simulink model "radar_simulation"  (R2022a)
settings: Solver=VariableStepAuto  StartTime=0.0  StopTime=10  RelTol=1e-3
model workspace (MAT data in the model file):
  Antenna_Aperture = Simulink.Parameter
  Antenna_Aperture.Value = 2.025e-05
  Antenna_Aperture.DataType = 'auto'
  Antenna_Aperture.Min = 0
  Antenna_Aperture.DocUnits = 'm^2'
  Antenna_Aperture.Complexity = 'real'
  Antenna_Aperture.Dimensions = [1 1]
  Center_Frequency = Simulink.Parameter
  Center_Frequency.Value = 60000000000
  Center_Frequency.DataType = 'auto'
  Center_Frequency.Min = 60000000000
  Center_Frequency.Max = 64000000000
  Center_Frequency.DocUnits = 'Hz'
  Center_Frequency.Complexity = 'real'
  Center_Frequency.Dimensions = [1 1]
  Max_Range = Simulink.Parameter
  Max_Range.Value = 100
  Max_Range.DataType = 'auto'
  Max_Range.Min = 0
  Max_Range.DocUnits = 'm'
  Max_Range.Complexity = 'real'
  Max_Range.Dimensions = [1 1]
  Sample_Rate = Simulink.Parameter
  Sample_Rate.Value = 16000000
  Sample_Rate.DataType = 'auto'
  Sample_Rate.Min = 0
  Sample_Rate.DocUnits = 'Hz'
  Sample_Rate.Complexity = 'real'
  Sample_Rate.Dimensions = [1 1]
  Samples_Per_CPI = Simulink.Parameter
  Samples_Per_CPI.Value = Simulink.data.Expression
  Samples_Per_CPI.Value.ExpressionString = "Samples_Per_Sweep * Sweeps_Per_CPI"
  Samples_Per_CPI.DataType = 'auto'
  Samples_Per_CPI.Complexity = 'real'
  Samples_Per_CPI.Dimensions = -1
  Samples_Per_Sweep = Simulink.Parameter
  Samples_Per_Sweep.Value = Simulink.data.Expression
  Samples_Per_Sweep.Value.ExpressionString = "Sample_Rate * Sweep_Interval"
  Samples_Per_Sweep.DataType = 'auto'
  Samples_Per_Sweep.Complexity = 'real'
  Samples_Per_Sweep.Dimensions = -1
  Sweep_Bandwidth = Simulink.Parameter
  Sweep_Bandwidth.Value = 135000000
  Sweep_Bandwidth.DataType = 'auto'
  Sweep_Bandwidth.Min = 0
  Sweep_Bandwidth.DocUnits = 'Hz'
  Sweep_Bandwidth.Complexity = 'real'
  Sweep_Bandwidth.Dimensions = [1 1]
  Sweep_Interval = Simulink.Parameter
  Sweep_Interval.Value = 4.5e-05
  Sweep_Interval.DataType = 'auto'
  Sweep_Interval.DocUnits = 's'
  Sweep_Interval.Complexity = 'real'
  Sweep_Interval.Dimensions = [1 1]
  Sweeps_Per_CPI = Simulink.Parameter
  Sweeps_Per_CPI.Value = 128
  Sweeps_Per_CPI.DataType = 'auto'
  Sweeps_Per_CPI.Complexity = 'real'
  Sweeps_Per_CPI.Dimensions = [1 1]
undefined symbols (not defined in the file or in its folder): aperture2gain, freq2wavelen, physconst
libraries: phasedenvlib x4, phaseddetectlib x2, phasedtxrxlib x2, phasedwavlib x1
settings Model: SimulationMode=accelerator  Creator=mhatch  LastModifiedBy=mhatch
settings SolverCC: DecoupledContinuousIntegration=on  MinimalZcImpactIntegration=on
settings DebuggingCC: ReadBeforeWriteMsg=DisableAll  WriteAfterWriteMsg=DisableAll  WriteAfterReadMsg=DisableAll  MultiTaskDSMMsg=none  AllowSymbolicDim=off
settings ModelReferenceCC: UpdateModelReferenceTargets=IfOutOfDate
settings SFSimCC: SFSimEcho=off

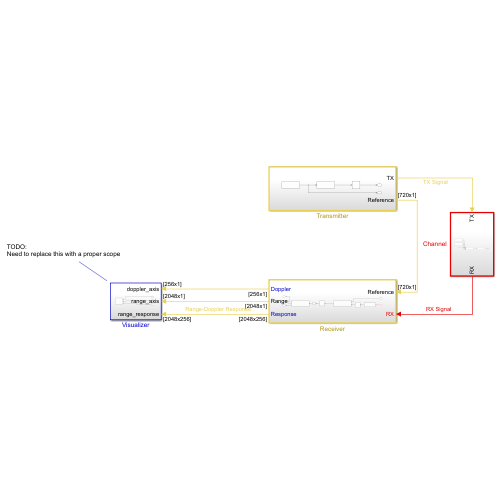
[thumbnail: Simulink's stored preview of the top-level diagram]
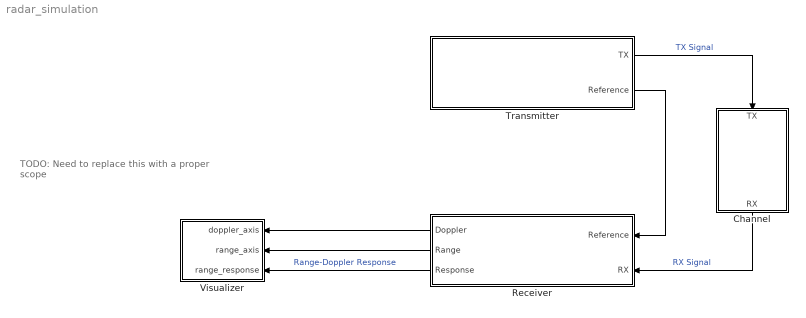
== system radar_simulation ==
  note: TODO:
      | Need to replace this with a proper scope
  Channel : Subsystem  TreatAsAtomicUnit=on
  Receiver : Subsystem  TreatAsAtomicUnit=on
  Transmitter : Subsystem  TreatAsAtomicUnit=on
  Visualizer : Subsystem
  wires:
  Transmitter/1(TX) -> Channel/1(TX)  "TX Signal"
  Channel/1(RX) -> Receiver/2(RX)  "RX Signal"
  Receiver/1(Doppler) -> Visualizer/1(doppler_axis)
  Receiver/2(Range) -> Visualizer/2(range_axis)
  Receiver/3(Response) -> Visualizer/3(range_response)  "Range-Doppler Response"
  Transmitter/2(Reference) -> Receiver/1(Reference)

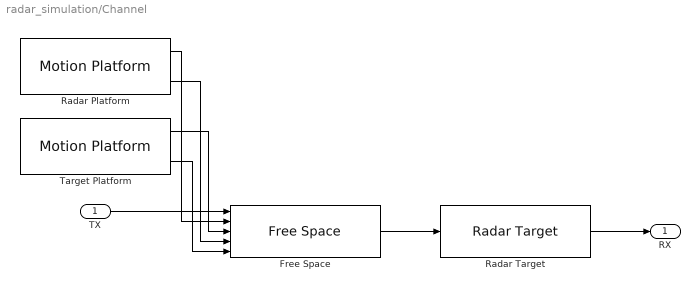
== system radar_simulation/Channel ==
  TX : Inport
  Free Space : phasedenvlib/Free Space  PropagationSpeed=physconst( 'LightSpeed' )  OperatingFrequency=Center_Frequency  TwoWayPropagation=on  SampleRateFromInputCheckbox=on  SampleRate=Sample_Rate  MaximumDistanceSource=Property  MaximumDistance=100  MaximumNumInputSamplesSource=Auto  MaximumNumInputSamples=1000  SimulateUsing=Code generation
      settings: SourceProductBaseCode=AR
  Radar Platform : phasedenvlib/Motion Platform  MotionModel=Velocity  InitialPosition=[ 0; 0; 0.5 ]  InitialVelocity=[ 0; 0; 0 ]  VelocitySource=Property  Velocity=[0; 0; 0]  AccelerationSource=Property  Acceleration=[0;0;0]  CustomTrajectory=[ 0, 0, 0, 0, 0, 0, 0; 1, 0, 0, 0, 0, 0, 0 ]  ScanMode=None  InitialScanAngle=0  AzimuthSpan=[ -60, 60 ]  AzimuthScanRate=10  InitialOrientationAxes=eye( 3 )  OrientationAxesOutputPort=off  ElapsedTimeSource=Auto  SampleRateFromInputCheckbox=on  SampleRate=1e6  SimulateUsing=Code generation
      settings: SourceProductBaseCode=AR
  Radar Target : phasedenvlib/Radar Target  EnablePolarization=off  Mode=Monostatic  MeanRCSSource=Property  ScatteringMatrixSource=Property  MeanRCS=min(pow2db(20), 0.1)  ScatteringMatrix=eye( 2 )  Model=Nonfluctuating  PropagationSpeed=physconst( 'LightSpeed' )  OperatingFrequency=Center_Frequency  SeedSource=Auto  Seed=0  SimulateUsing=Code generation
      settings: SourceProductBaseCode=AR
  Target Platform : phasedenvlib/Motion Platform  MotionModel=Velocity  InitialPosition=[ 20; 0; 0.5 ]  InitialVelocity=[ 0; 0; 0 ]  VelocitySource=Property  Velocity=[5; 0; 0]  AccelerationSource=Property  Acceleration=[0;0;0]  CustomTrajectory=[ 0, 0, 0, 0, 0, 0, 0; 1, 0, 0, 0, 0, 0, 0 ]  ScanMode=None  InitialScanAngle=0  AzimuthSpan=[ -60, 60 ]  AzimuthScanRate=10  InitialOrientationAxes=eye( 3 )  OrientationAxesOutputPort=off  ElapsedTimeSource=Auto  SampleRateFromInputCheckbox=on  SampleRate=1e6  SimulateUsing=Code generation
      settings: SourceProductBaseCode=AR
  RX : Outport
  wires:
  Radar Platform/1 -> Free Space/2
  Radar Platform/2 -> Free Space/4
  Target Platform/2 -> Free Space/5
  Target Platform/1 -> Free Space/3
  TX/1 -> Free Space/1
  Free Space/1 -> Radar Target/1
  Radar Target/1 -> RX/1

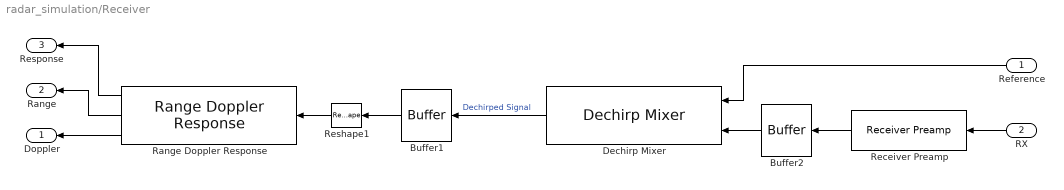
== system radar_simulation/Receiver ==
  Reference : Inport
  RX : Inport  Port=2
  Buffer1 : Buffer  N=Samples_Per_CPI  OutputFrames=off
  Buffer2 : Buffer  N=Samples_Per_Sweep  OutputFrames=off
  Dechirp Mixer : phaseddetectlib/Dechirp Mixer
      settings: SourceProductBaseCode=AR
  Range Doppler Response : phaseddetectlib/Range Doppler Response  RangeMethod=FFT  PropagationSpeed=physconst( 'lightspeed' )  SampleRateFromInputCheckbox=off  SampleRate=Sample_Rate  SweepSlope=Sweep_Bandwidth / Sweep_Interval  DechirpInput=off  RangeFFTLengthSource=Property  RangeFFTLength=2048  RangeWindow=None  RangeSidelobeAttenuation=30  CustomRangeWindow=@hamming  ReferenceRangeCentered=on  ReferenceRange=0  MaximumNumInputSamplesSource=Auto  MaximumNumInputSamples=100  PRFSource=Auto  PRF=10e3  DopplerFFTLengthSource=Property  DopplerFFTLength=256  DopplerWindow=None  DopplerSidelobeAttenuation=30  CustomDopplerWindow=@hamming  DopplerOutput=Speed  OperatingFrequency=Center_Frequency  SimulateUsing=Code generation
      settings: SourceProductBaseCode=AR
  Receiver Preamp : phasedtxrxlib/Receiver Preamp  Gain=15 + aperture2gain(Antenna_Aperture, freq2wavelen(Center_Frequency, physconst( 'LightSpeed')))  LossFactor=0  NoiseMethod=Noise temperature  NoiseFigure=4.5  ReferenceTemperature=290  SampleRateFromInputCheckbox=on  SampleRate=1e6  NoisePower=0  EnableInputPort=off  PhaseNoiseInputPort=off  SeedSource=Auto  Seed=0  SimulateUsing=Code generation
      settings: SourceProductBaseCode=AR
  Reshape1 : Reshape  OutputDimensionality=Customize  OutputDimensions=[Samples_Per_Sweep Sweeps_Per_CPI]
  Doppler : Outport
  Range : Outport  Port=2
  Response : Outport  Port=3
  wires:
  Buffer1/1 -> Reshape1/1
  Reference/1 -> Dechirp Mixer/1
  RX/1 -> Receiver Preamp/1
  Reshape1/1 -> Range Doppler Response/1
  Dechirp Mixer/1 -> Buffer1/1  "Dechirped Signal"
  Buffer2/1 -> Dechirp Mixer/2
  Receiver Preamp/1 -> Buffer2/1
  Range Doppler Response/3 -> Doppler/1
  Range Doppler Response/1 -> Response/1
  Range Doppler Response/2 -> Range/1

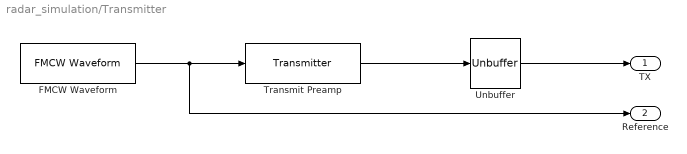
== system radar_simulation/Transmitter ==
  FMCW Waveform : phasedwavlib/FMCW Waveform  SampleRate=Sample_Rate  SweepTime=Sweep_Interval  SweepBandwidth=Sweep_Bandwidth  SweepDirection=Up  SweepInterval=Positive  OutputFormat=Sweeps  NumSamples=100  NumSweeps=1  SimulateUsing=Code generation
      settings: SourceProductBaseCode=AR
  Transmit Preamp : phasedtxrxlib/Transmitter  PeakPower=db2pow(10)  Gain=9 + aperture2gain(Antenna_Aperture, freq2wavelen(Center_Frequency, physconst( 'LightSpeed' )))  LossFactor=0  InUseOutputPort=off  CoherentOnTransmit=on  PhaseNoiseOutputPort=off  SeedSource=Auto  Seed=0  SimulateUsing=Code generation
      settings: SourceProductBaseCode=AR
  Unbuffer : Unbuffer
  TX : Outport
  Reference : Outport  Port=2
  wires:
  Transmit Preamp/1 -> Unbuffer/1
  Unbuffer/1 -> TX/1
  FMCW Waveform/1 -> Reference/1, Transmit Preamp/1

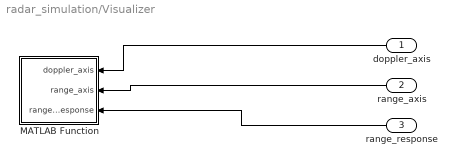
== system radar_simulation/Visualizer ==
  doppler_axis : Inport
  range_axis : Inport  Port=2
  range_response : Inport  Port=3
  MATLAB Function : MATLAB Function  TreatAsAtomicUnit=on
  wires:
  doppler_axis/1 -> MATLAB Function/1(doppler_axis)
  range_axis/1 -> MATLAB Function/2(range_axis)
  range_response/1 -> MATLAB Function/3(range_response)

== matlab function radar_simulation/Visualizer/MATLAB Function ==
  data: doppler_axis input; range_axis input; range_response input
function fcn(doppler_axis, range_axis, range_response)

coder.extrinsic('imagesc');

imagesc(doppler_axis, range_axis, mag2db(abs(range_response)));
xlabel('Speed (m/s)');
ylabel('Range (m)');
title('Range-Doppler Map');

end
